simulink model "RaibertControl"  (R2022a)
settings: Solver=ode4  StartTime=0.0  StopTime=10  FixedStep=1/1000  RelTol=1e-3  AbsTol=1e-3  EnableMultiTasking=on
undefined symbols (not defined in the file or in its folder): Carrier, N, Ring, T, X, Y, Z
libraries: sm_lib x133, nesl_utility x25, Multibody_Parts_Lib x4, fl_lib x4
(part 7 of 7)

== matlab function RaibertControl/Final/Impedance Control1/to_dPolar ==
  data: theta1 input; theta2 input; dr output; dphi output; dtheta1 input; dtheta2 input
function [dr,dphi] = Velocity(theta1,theta2,dtheta1,dtheta2)
%VELOCITY
%    [DR,DPHI] = VELOCITY(THETA1,THETA2,DTHETA1,DTHETA2)

%    This function was generated by the Symbolic Math Toolbox version 8.6.
%    17-May-2022 09:32:08

dr = dtheta1.*(sin(acos(sqrt((sin(theta1-pi./2.0).*(7.0./4.0e+1)+sin(theta2+pi./2.0).*(7.0./4.0e+1)).^2+abs(cos(theta1-pi./2.0).*(7.0./4.0e+1)+cos(theta2+pi./2.0).*(7.0./4.0e+1)+3.0./2.5e+1).^2).*(5.0./3.0))+atan2(sin(theta1-pi./2.0).*(-7.0./4.0e+1)-sin(theta2+pi./2.0).*(7.0./4.0e+1),abs(cos(theta1-pi./2.0).*(7.0./4.0e+1)+cos(theta2+pi./2.0).*(7.0./4.0e+1)+3.0./2.5e+1))+6.012387278395987e-2).*(1.0./sqrt((sin(theta1-pi./2.0).*(7.0./4.0e+1)+sin(theta2+pi./2.0).*(7.0./4.0e+1)).^2+abs(cos(theta1-pi./2.0).*(7.0./4.0e+1)+cos(theta2+pi./2.0).*(7.0./4.0e+1)+3.0./2.5e+1).^2).*(cos(theta1-pi./2.0).*(sin(theta1-pi./2.0).*(7.0./4.0e+1)+sin(theta2+pi./2.0).*(7.0./4.0e+1)).*(7.0./2.0e+1)-abs(cos(theta1-pi./2.0).*(7.0./4.0e+1)+cos(theta2+pi./2.0).*(7.0./4.0e+1)+3.0./2.5e+1).*sign(cos(theta1-pi./2.0).*(7.0./4.0e+1)+cos(theta2+pi./2.0).*(7.0./4.0e+1)+3.0./2.5e+1).*sin(theta1-pi./2.0).*(7.0./2.0e+1)).*1.0./sqrt((sin(theta1-pi./2.0).*(7.0./4.0e+1)+sin(theta2+pi./2.0).*(7.0./4.0e+1)).^2.*(-2.5e+1./9.0)-abs(cos(theta1-pi./2.0).*(7.0./4.0e+1)+cos(theta2+pi./2.0).*(7.0./4.0e+1)+3.0./2.5e+1).^2.*(2.5e+1./9.0)+1.0).*(5.0./6.0)+(abs(cos(theta1-pi./2.0).*(7.0./4.0e+1)+cos(theta2+pi./2.0).*(7.0./4.0e+1)+3.0./2.5e+1).^2.*((cos(theta1-pi./2.0).*(7.0./4.0e+1))./abs(cos(theta1-pi./2.0).*(7.0./4.0e+1)+cos(theta2+pi./2.0).*(7.0./4.0e+1)+3.0./2.5e+1)+1.0./abs(cos(theta1-pi./2.0).*(7.0./4.0e+1)+cos(theta2+pi./2.0).*(7.0./4.0e+1)+3.0./2.5e+1).^2.*sign(cos(theta1-pi./2.0).*(7.0./4.0e+1)+cos(theta2+pi./2.0).*(7.0./4.0e+1)+3.0./2.5e+1).*sin(theta1-pi./2.0).*(sin(theta1-pi./2.0).*(7.0./4.0e+1)+sin(theta2+pi./2.0).*(7.0./4.0e+1)).*(7.0./4.0e+1)))./((sin(theta1-pi./2.0).*(7.0./4.0e+1)+sin(theta2+pi./2.0).*(7.0./4.0e+1)).^2+abs(cos(theta1-pi./2.0).*(7.0./4.0e+1)+cos(theta2+pi./2.0).*(7.0./4.0e+1)+3.0./2.5e+1).^2)).*(cos(acos(sqrt((sin(theta1-pi./2.0).*(7.0./4.0e+1)+sin(theta2+pi./2.0).*(7.0./4.0e+1)).^2+abs(cos(theta1-pi./2.0).*(7.0./4.0e+1)+cos(theta2+pi./2.0).*(7.0./4.0e+1)+3.0./2.5e+1).^2).*(5.0./3.0))+atan2(sin(theta1-pi./2.0).*(-7.0./4.0e+1)-sin(theta2+pi./2.0).*(7.0./4.0e+1),abs(cos(theta1-pi./2.0).*(7.0./4.0e+1)+cos(theta2+pi./2.0).*(7.0./4.0e+1)+3.0./2.5e+1))+6.012387278395987e-2).*(-3.328470665197855e-1)+cos(theta2+pi./2.0).*(7.0./4.0e+1)+3.0./5.0e+1).*6.65694133039571e-1+cos(acos(sqrt((sin(theta1-pi./2.0).*(7.0./4.0e+1)+sin(theta2+pi./2.0).*(7.0./4.0e+1)).^2+abs(cos(theta1-pi./2.0).*(7.0./4.0e+1)+cos(theta2+pi./2.0).*(7.0./4.0e+1)+3.0./2.5e+1).^2).*(5.0./3.0))+atan2(sin(theta1-pi./2.0).*(-7.0./4.0e+1)-sin(theta2+pi./2.0).*(7.0./4.0e+1),abs(cos(theta1-pi./2.0).*(7.0./4.0e+1)+cos(theta2+pi./2.0).*(7.0./4.0e+1)+3.0./2.5e+1))+6.012387278395987e-2).*(sin(acos(sqrt((sin(theta1-pi./2.0).*(7.0./4.0e+1)+sin(theta2+pi./2.0).*(7.0./4.0e+1)).^2+abs(cos(theta1-pi./2.0).*(7.0./4.0e+1)+cos(theta2+pi./2.0).*(7.0./4.0e+1)+3.0./2.5e+1).^2).*(5.0./3.0))+atan2(sin(theta1-pi./2.0).*(-7.0./4.0e+1)-sin(theta2+pi./2.0).*(7.0./4.0e+1),abs(cos(theta1-pi./2.0).*(7.0./4.0e+1)+cos(theta2+pi./2.0).*(7.0./4.0e+1)+3.0./2.5e+1))+6.012387278395987e-2).*3.328470665197855e-1+sin(theta2+pi./2.0).*(7.0./4.0e+1)).*(1.0./sqrt((sin(theta1-pi./2.0).*(7.0./4.0e+1)+sin(theta2+pi./2.0).*(7.0./4.0e+1)).^2+abs(cos(theta1-pi./2.0).*(7.0./4.0e+1)+cos(theta2+pi./2.0).*(7.0./4.0e+1)+3.0./2.5e+1).^2).*(cos(theta1-pi./2.0).*(sin(theta1-pi./2.0).*(7.0./4.0e+1)+sin(theta2+pi./2.0).*(7.0./4.0e+1)).*(7.0./2.0e+1)-abs(cos(theta1-pi./2.0).*(7.0./4.0e+1)+cos(theta2+pi./2.0).*(7.0./4.0e+1)+3.0./2.5e+1).*sign(cos(theta1-pi./2.0).*(7.0./4.0e+1)+cos(theta2+pi./2.0).*(7.0./4.0e+1)+3.0./2.5e+1).*sin(theta1-pi./2.0).*(7.0./2.0e+1)).*1.0./sqrt((sin(theta1-pi./2.0).*(7.0./4.0e+1)+sin(theta2+pi./2.0).*(7.0./4.0e+1)).^2.*(-2.5e+1./9.0)-abs(cos(theta1-pi./2.0).*(7.0./4.0e+1)+cos(theta2+pi./2.0).*(7.0./4.0e+1)+3.0./2.5e+1).^2.*(2.5e+1./9.0)+1.0).*(5.0./6.0)+(abs(cos(theta1-pi./2.0).*(7.0./4.0e+1)+cos(theta2+pi./2.0).*(7.0./4.0e+1)+3.0./2.5e+1).^2.*((cos(theta1-pi./2.0).*(7.0./4.0e+1))./abs(cos(theta1-pi./2.0).*(7.0./4.0e+1)+cos(theta2+pi./2.0).*(7.0./4.0e+1)+3.0./2.5e+1)+1.0./abs(cos(theta1-pi./2.0).*(7.0./4.0e+1)+cos(theta2+pi./2.0).*(7.0./4.0e+1)+3.0./2.5e+1).^2.*sign(cos(theta1-pi./2.0).*(7.0./4.0e+1)+cos(theta2+pi./2.0).*(7.0./4.0e+1)+3.0./2.5e+1).*sin(theta1-pi./2.0).*(sin(theta1-pi./2.0).*(7.0./4.0e+1)+sin(theta2+pi./2.0).*(7.0./4.0e+1)).*(7.0./4.0e+1)))./((sin(theta1-pi./2.0).*(7.0./4.0e+1)+sin(theta2+pi./2.0).*(7.0./4.0e+1)).^2+abs(cos(theta1-pi./2.0).*(7.0./4.0e+1)+cos(theta2+pi./2.0).*(7.0./4.0e+1)+3.0./2.5e+1).^2)).*6.65694133039571e-1).*1.0./sqrt((cos(acos(sqrt((sin(theta1-pi./2.0).*(7.0./4.0e+1)+sin(theta2+pi./2.0).*(7.0./4.0e+1)).^2+abs(cos(theta1-pi./2.0).*(7.0./4.0e+1)+cos(theta2+pi./2.0).*(7.0./4.0e+1)+3.0./2.5e+1).^2).*(5.0./3.0))+atan2(sin(theta1-pi./2.0).*(-7.0./4.0e+1)-sin(theta2+pi./2.0).*(7.0./4.0e+1),abs(cos(theta1-pi./2.0).*(7.0./4.0e+1)+cos(theta2+pi./2.0).*(7.0./4.0e+1)+3.0./2.5e+1))+6.012387278395987e-2).*(-3.328470665197855e-1)+cos(theta2+pi./2.0).*(7.0./4.0e+1)+3.0./5.0e+1).^2+(sin(acos(sqrt((sin(theta1-pi./2.0).*(7.0./4.0e+1)+sin(theta2+pi./2.0).*(7.0./4.0e+1)).^2+abs(cos(theta1-pi./2.0).*(7.0./4.0e+1)+cos(theta2+pi./2.0).*(7.0./4.0e+1)+3.0./2.5e+1).^2).*(5.0./3.0))+atan2(sin(theta1-pi./2.0).*(-7.0./4.0e+1)-sin(theta2+pi./2.0).*(7.0./4.0e+1),abs(cos(theta1-pi./2.0).*(7.0./4.0e+1)+cos(theta2+pi./2.0).*(7.0./4.0e+1)+3.0./2.5e+1))+6.012387278395987e-2).*3.328470665197855e-1+sin(theta2+pi./2.0).*(7.0./4.0e+1)).^2).*(-1.0./2.0)+(dtheta2.*((sin(acos(sqrt((sin(theta1-pi./2.0).*(7.0./4.0e+1)+sin(theta2+pi./2.0).*(7.0./4.0e+1)).^2+abs(cos(theta1-pi./2.0).*(7.0./4.0e+1)+cos(theta2+pi./2.0).*(7.0./4.0e+1)+3.0./2.5e+1).^2).*(5.0./3.0))+atan2(sin(theta1-pi./2.0).*(-7.0./4.0e+1)-sin(theta2+pi./2.0).*(7.0./4.0e+1),abs(cos(theta1-pi./2.0).*(7.0./4.0e+1)+cos(theta2+pi./2.0).*(7.0./4.0e+1)+3.0./2.5e+1))+6.012387278395987e-2).*3.328470665197855e-1+sin(theta2+pi./2.0).*(7.0./4.0e+1)).*(cos(theta2+pi./2.0).*(7.0./4.0e+1)-cos(acos(sqrt((sin(theta1-pi./2.0).*(7.0./4.0e+1)+sin(theta2+pi./2.0).*(7.0./4.0e+1)).^2+abs(cos(theta1-pi./2.0).*(7.0./4.0e+1)+cos(theta2+pi./2.0).*(7.0./4.0e+1)+3.0./2.5e+1).^2).*(5.0./3.0))+atan2(sin(theta1-pi./2.0).*(-7.0./4.0e+1)-sin(theta2+pi./2.0).*(7.0./4.0e+1),abs(cos(theta1-pi./2.0).*(7.0./4.0e+1)+cos(theta2+pi./2.0).*(7.0./4.0e+1)+3.0./2.5e+1))+6.012387278395987e-2).*(1.0./sqrt((sin(theta1-pi./2.0).*(7.0./4.0e+1)+sin(theta2+pi./2.0).*(7.0./4.0e+1)).^2+abs(cos(theta1-pi./2.0).*(7.0./4.0e+1)+cos(theta2+pi./2.0).*(7.0./4.0e+1)+3.0./2.5e+1).^2).*(cos(theta2+pi./2.0).*(sin(theta1-pi./2.0).*(7.0./4.0e+1)+sin(theta2+pi./2.0).*(7.0./4.0e+1)).*(7.0./2.0e+1)-abs(cos(theta1-pi./2.0).*(7.0./4.0e+1)+cos(theta2+pi./2.0).*(7.0./4.0e+1)+3.0./2.5e+1).*sign(cos(theta1-pi./2.0).*(7.0./4.0e+1)+cos(theta2+pi./2.0).*(7.0./4.0e+1)+3.0./2.5e+1).*sin(theta2+pi./2.0).*(7.0./2.0e+1)).*1.0./sqrt((sin(theta1-pi./2.0).*(7.0./4.0e+1)+sin(theta2+pi./2.0).*(7.0./4.0e+1)).^2.*(-2.5e+1./9.0)-abs(cos(theta1-pi./2.0).*(7.0./4.0e+1)+cos(theta2+pi./2.0).*(7.0./4.0e+1)+3.0./2.5e+1).^2.*(2.5e+1./9.0)+1.0).*(5.0./6.0)+(abs(cos(theta1-pi./2.0).*(7.0./4.0e+1)+cos(theta2+pi./2.0).*(7.0./4.0e+1)+3.0./2.5e+1).^2.*((cos(theta2+pi./2.0).*(7.0./4.0e+1))./abs(cos(theta1-pi./2.0).*(7.0./4.0e+1)+cos(theta2+pi./2.0).*(7.0./4.0e+1)+3.0./2.5e+1)+1.0./abs(cos(theta1-pi./2.0).*(7.0./4.0e+1)+cos(theta2+pi./2.0).*(7.0./4.0e+1)+3.0./2.5e+1).^2.*sign(cos(theta1-pi./2.0).*(7.0./4.0e+1)+cos(theta2+pi./2.0).*(7.0./4.0e+1)+3.0./2.5e+1).*sin(theta2+pi./2.0).*(sin(theta1-pi./2.0).*(7.0./4.0e+1)+sin(theta2+pi./2.0).*(7.0./4.0e+1)).*(7.0./4.0e+1)))./((sin(theta1-pi./2.0).*(7.0./4.0e+1)+sin(theta2+pi./2.0).*(7.0./4.0e+1)).^2+abs(cos(theta1-pi./2.0).*(7.0./4.0e+1)+cos(theta2+pi./2.0).*(7.0./4.0e+1)+3.0./2.5e+1).^2)).*3.328470665197855e-1).*2.0-(sin(theta2+pi./2.0).*(7.0./4.0e+1)+sin(acos(sqrt((sin(theta1-pi./2.0).*(7.0./4.0e+1)+sin(theta2+pi./2.0).*(7.0./4.0e+1)).^2+abs(cos(theta1-pi./2.0).*(7.0./4.0e+1)+cos(theta2+pi./2.0).*(7.0./4.0e+1)+3.0./2.5e+1).^2).*(5.0./3.0))+atan2(sin(theta1-pi./2.0).*(-7.0./4.0e+1)-sin(theta2+pi./2.0).*(7.0./4.0e+1),abs(cos(theta1-pi./2.0).*(7.0./4.0e+1)+cos(theta2+pi./2.0).*(7.0./4.0e+1)+3.0./2.5e+1))+6.012387278395987e-2).*(1.0./sqrt((sin(theta1-pi./2.0).*(7.0./4.0e+1)+sin(theta2+pi./2.0).*(7.0./4.0e+1)).^2+abs(cos(theta1-pi./2.0).*(7.0./4.0e+1)+cos(theta2+pi./2.0).*(7.0./4.0e+1)+3.0./2.5e+1).^2).*(cos(theta2+pi./2.0).*(sin(theta1-pi./2.0).*(7.0./4.0e+1)+sin(theta2+pi./2.0).*(7.0./4.0e+1)).*(7.0./2.0e+1)-abs(cos(theta1-pi./2.0).*(7.0./4.0e+1)+cos(theta2+pi./2.0).*(7.0./4.0e+1)+3.0./2.5e+1).*sign(cos(theta1-pi./2.0).*(7.0./4.0e+1)+cos(theta2+pi./2.0).*(7.0./4.0e+1)+3.0./2.5e+1).*sin(theta2+pi./2.0).*(7.0./2.0e+1)).*1.0./sqrt((sin(theta1-pi./2.0).*(7.0./4.0e+1)+sin(theta2+pi./2.0).*(7.0./4.0e+1)).^2.*(-2.5e+1./9.0)-abs(cos(theta1-pi./2.0).*(7.0./4.0e+1)+cos(theta2+pi./2.0).*(7.0./4.0e+1)+3.0./2.5e+1).^2.*(2.5e+1./9.0)+1.0).*(5.0./6.0)+(abs(cos(theta1-pi./2.0).*(7.0./4.0e+1)+cos(theta2+pi./2.0).*(7.0./4.0e+1)+3.0./2.5e+1).^2.*((cos(theta2+pi./2.0).*(7.0./4.0e+1))./abs(cos(theta1-pi./2.0).*(7.0./4.0e+1)+cos(theta2+pi./2.0).*(7.0./4.0e+1)+3.0./2.5e+1)+1.0./abs(cos(theta1-pi./2.0).*(7.0./4.0e+1)+cos(theta2+pi./2.0).*(7.0./4.0e+1)+3.0./2.5e+1).^2.*sign(cos(theta1-pi./2.0).*(7.0./4.0e+1)+cos(theta2+pi./2.0).*(7.0./4.0e+1)+3.0./2.5e+1).*sin(theta2+pi./2.0).*(sin(theta1-pi./2.0).*(7.0./4.0e+1)+sin(theta2+pi./2.0).*(7.0./4.0e+1)).*(7.0./4.0e+1)))./((sin(theta1-pi./2.0).*(7.0./4.0e+1)+sin(theta2+pi./2.0).*(7.0./4.0e+1)).^2+abs(cos(theta1-pi./2.0).*(7.0./4.0e+1)+cos(theta2+pi./2.0).*(7.0./4.0e+1)+3.0./2.5e+1).^2)).*3.328470665197855e-1).*(cos(acos(sqrt((sin(theta1-pi./2.0).*(7.0./4.0e+1)+sin(theta2+pi./2.0).*(7.0./4.0e+1)).^2+abs(cos(theta1-pi./2.0).*(7.0./4.0e+1)+cos(theta2+pi./2.0).*(7.0./4.0e+1)+3.0./2.5e+1).^2).*(5.0./3.0))+atan2(sin(theta1-pi./2.0).*(-7.0./4.0e+1)-sin(theta2+pi./2.0).*(7.0./4.0e+1),abs(cos(theta1-pi./2.0).*(7.0./4.0e+1)+cos(theta2+pi./2.0).*(7.0./4.0e+1)+3.0./2.5e+1))+6.012387278395987e-2).*(-3.328470665197855e-1)+cos(theta2+pi./2.0).*(7.0./4.0e+1)+3.0./5.0e+1).*2.0).*1.0./sqrt((cos(acos(sqrt((sin(theta1-pi./2.0).*(7.0./4.0e+1)+sin(theta2+pi./2.0).*(7.0./4.0e+1)).^2+abs(cos(theta1-pi./2.0).*(7.0./4.0e+1)+cos(theta2+pi./2.0).*(7.0./4.0e+1)+3.0./2.5e+1).^2).*(5.0./3.0))+atan2(sin(theta1-pi./2.0).*(-7.0./4.0e+1)-sin(theta2+pi./2.0).*(7.0./4.0e+1),abs(cos(theta1-pi./2.0).*(7.0./4.0e+1)+cos(theta2+pi./2.0).*(7.0./4.0e+1)+3.0./2.5e+1))+6.012387278395987e-2).*(-3.328470665197855e-1)+cos(theta2+pi./2.0).*(7.0./4.0e+1)+3.0./5.0e+1).^2+(sin(acos(sqrt((sin(theta1-pi./2.0).*(7.0./4.0e+1)+sin(theta2+pi./2.0).*(7.0./4.0e+1)).^2+abs(cos(theta1-pi./2.0).*(7.0./4.0e+1)+cos(theta2+pi./2.0).*(7.0./4.0e+1)+3.0./2.5e+1).^2).*(5.0./3.0))+atan2(sin(theta1-pi./2.0).*(-7.0./4.0e+1)-sin(theta2+pi./2.0).*(7.0./4.0e+1),abs(cos(theta1-pi./2.0).*(7.0./4.0e+1)+cos(theta2+pi./2.0).*(7.0./4.0e+1)+3.0./2.5e+1))+6.012387278395987e-2).*3.328470665197855e-1+sin(theta2+pi./2.0).*(7.0./4.0e+1)).^2))./2.0;
if nargout > 1
    dphi = (dtheta1.*((cos(acos(sqrt((sin(theta1-pi./2.0).*(7.0./4.0e+1)+sin(theta2+pi./2.0).*(7.0./4.0e+1)).^2+abs(cos(theta1-pi./2.0).*(7.0./4.0e+1)+cos(theta2+pi./2.0).*(7.0./4.0e+1)+3.0./2.5e+1).^2).*(5.0./3.0))+atan2(sin(theta1-pi./2.0).*(-7.0./4.0e+1)-sin(theta2+pi./2.0).*(7.0./4.0e+1),abs(cos(theta1-pi./2.0).*(7.0./4.0e+1)+cos(theta2+pi./2.0).*(7.0./4.0e+1)+3.0./2.5e+1))+6.012387278395987e-2).*(1.0./sqrt((sin(theta1-pi./2.0).*(7.0./4.0e+1)+sin(theta2+pi./2.0).*(7.0./4.0e+1)).^2+abs(cos(theta1-pi./2.0).*(7.0./4.0e+1)+cos(theta2+pi./2.0).*(7.0./4.0e+1)+3.0./2.5e+1).^2).*(cos(theta1-pi./2.0).*(sin(theta1-pi./2.0).*(7.0./4.0e+1)+sin(theta2+pi./2.0).*(7.0./4.0e+1)).*(7.0./2.0e+1)-abs(cos(theta1-pi./2.0).*(7.0./4.0e+1)+cos(theta2+pi./2.0).*(7.0./4.0e+1)+3.0./2.5e+1).*sign(cos(theta1-pi./2.0).*(7.0./4.0e+1)+cos(theta2+pi./2.0).*(7.0./4.0e+1)+3.0./2.5e+1).*sin(theta1-pi./2.0).*(7.0./2.0e+1)).*1.0./sqrt((sin(theta1-pi./2.0).*(7.0./4.0e+1)+sin(theta2+pi./2.0).*(7.0./4.0e+1)).^2.*(-2.5e+1./9.0)-abs(cos(theta1-pi./2.0).*(7.0./4.0e+1)+cos(theta2+pi./2.0).*(7.0./4.0e+1)+3.0./2.5e+1).^2.*(2.5e+1./9.0)+1.0).*(5.0./6.0)+(abs(cos(theta1-pi./2.0).*(7.0./4.0e+1)+cos(theta2+pi./2.0).*(7.0./4.0e+1)+3.0./2.5e+1).^2.*((cos(theta1-pi./2.0).*(7.0./4.0e+1))./abs(cos(theta1-pi./2.0).*(7.0./4.0e+1)+cos(theta2+pi./2.0).*(7.0./4.0e+1)+3.0./2.5e+1)+1.0./abs(cos(theta1-pi./2.0).*(7.0./4.0e+1)+cos(theta2+pi./2.0).*(7.0./4.0e+1)+3.0./2.5e+1).^2.*sign(cos(theta1-pi./2.0).*(7.0./4.0e+1)+cos(theta2+pi./2.0).*(7.0./4.0e+1)+3.0./2.5e+1).*sin(theta1-pi./2.0).*(sin(theta1-pi./2.0).*(7.0./4.0e+1)+sin(theta2+pi./2.0).*(7.0./4.0e+1)).*(7.0./4.0e+1)))./((sin(theta1-pi./2.0).*(7.0./4.0e+1)+sin(theta2+pi./2.0).*(7.0./4.0e+1)).^2+abs(cos(theta1-pi./2.0).*(7.0./4.0e+1)+cos(theta2+pi./2.0).*(7.0./4.0e+1)+3.0./2.5e+1).^2)).*3.328470665197855e-1)./(cos(acos(sqrt((sin(theta1-pi./2.0).*(7.0./4.0e+1)+sin(theta2+pi./2.0).*(7.0./4.0e+1)).^2+abs(cos(theta1-pi./2.0).*(7.0./4.0e+1)+cos(theta2+pi./2.0).*(7.0./4.0e+1)+3.0./2.5e+1).^2).*(5.0./3.0))+atan2(sin(theta1-pi./2.0).*(-7.0./4.0e+1)-sin(theta2+pi./2.0).*(7.0./4.0e+1),abs(cos(theta1-pi./2.0).*(7.0./4.0e+1)+cos(theta2+pi./2.0).*(7.0./4.0e+1)+3.0./2.5e+1))+6.012387278395987e-2).*(-3.328470665197855e-1)+cos(theta2+pi./2.0).*(7.0./4.0e+1)+3.0./5.0e+1)-sin(acos(sqrt((sin(theta1-pi./2.0).*(7.0./4.0e+1)+sin(theta2+pi./2.0).*(7.0./4.0e+1)).^2+abs(cos(theta1-pi./2.0).*(7.0./4.0e+1)+cos(theta2+pi./2.0).*(7.0./4.0e+1)+3.0./2.5e+1).^2).*(5.0./3.0))+atan2(sin(theta1-pi./2.0).*(-7.0./4.0e+1)-sin(theta2+pi./2.0).*(7.0./4.0e+1),abs(cos(theta1-pi./2.0).*(7.0./4.0e+1)+cos(theta2+pi./2.0).*(7.0./4.0e+1)+3.0./2.5e+1))+6.012387278395987e-2).*(sin(acos(sqrt((sin(theta1-pi./2.0).*(7.0./4.0e+1)+sin(theta2+pi./2.0).*(7.0./4.0e+1)).^2+abs(cos(theta1-pi./2.0).*(7.0./4.0e+1)+cos(theta2+pi./2.0).*(7.0./4.0e+1)+3.0./2.5e+1).^2).*(5.0./3.0))+atan2(sin(theta1-pi./2.0).*(-7.0./4.0e+1)-sin(theta2+pi./2.0).*(7.0./4.0e+1),abs(cos(theta1-pi./2.0).*(7.0./4.0e+1)+cos(theta2+pi./2.0).*(7.0./4.0e+1)+3.0./2.5e+1))+6.012387278395987e-2).*3.328470665197855e-1+sin(theta2+pi./2.0).*(7.0./4.0e+1)).*(1.0./sqrt((sin(theta1-pi./2.0).*(7.0./4.0e+1)+sin(theta2+pi./2.0).*(7.0./4.0e+1)).^2+abs(cos(theta1-pi./2.0).*(7.0./4.0e+1)+cos(theta2+pi./2.0).*(7.0./4.0e+1)+3.0./2.5e+1).^2).*(cos(theta1-pi./2.0).*(sin(theta1-pi./2.0).*(7.0./4.0e+1)+sin(theta2+pi./2.0).*(7.0./4.0e+1)).*(7.0./2.0e+1)-abs(cos(theta1-pi./2.0).*(7.0./4.0e+1)+cos(theta2+pi./2.0).*(7.0./4.0e+1)+3.0./2.5e+1).*sign(cos(theta1-pi./2.0).*(7.0./4.0e+1)+cos(theta2+pi./2.0).*(7.0./4.0e+1)+3.0./2.5e+1).*sin(theta1-pi./2.0).*(7.0./2.0e+1)).*1.0./sqrt((sin(theta1-pi./2.0).*(7.0./4.0e+1)+sin(theta2+pi./2.0).*(7.0./4.0e+1)).^2.*(-2.5e+1./9.0)-abs(cos(theta1-pi./2.0).*(7.0./4.0e+1)+cos(theta2+pi./2.0).*(7.0./4.0e+1)+3.0./2.5e+1).^2.*(2.5e+1./9.0)+1.0).*(5.0./6.0)+(abs(cos(theta1-pi./2.0).*(7.0./4.0e+1)+cos(theta2+pi./2.0).*(7.0./4.0e+1)+3.0./2.5e+1).^2.*((cos(theta1-pi./2.0).*(7.0./4.0e+1))./abs(cos(theta1-pi./2.0).*(7.0./4.0e+1)+cos(theta2+pi./2.0).*(7.0./4.0e+1)+3.0./2.5e+1)+1.0./abs(cos(theta1-pi./2.0).*(7.0./4.0e+1)+cos(theta2+pi./2.0).*(7.0./4.0e+1)+3.0./2.5e+1).^2.*sign(cos(theta1-pi./2.0).*(7.0./4.0e+1)+cos(theta2+pi./2.0).*(7.0./4.0e+1)+3.0./2.5e+1).*sin(theta1-pi./2.0).*(sin(theta1-pi./2.0).*(7.0./4.0e+1)+sin(theta2+pi./2.0).*(7.0./4.0e+1)).*(7.0./4.0e+1)))./((sin(theta1-pi./2.0).*(7.0./4.0e+1)+sin(theta2+pi./2.0).*(7.0./4.0e+1)).^2+abs(cos(theta1-pi./2.0).*(7.0./4.0e+1)+cos(theta2+pi./2.0).*(7.0./4.0e+1)+3.0./2.5e+1).^2)).*1.0./(cos(acos(sqrt((sin(theta1-pi./2.0).*(7.0./4.0e+1)+sin(theta2+pi./2.0).*(7.0./4.0e+1)).^2+abs(cos(theta1-pi./2.0).*(7.0./4.0e+1)+cos(theta2+pi./2.0).*(7.0./4.0e+1)+3.0./2.5e+1).^2).*(5.0./3.0))+atan2(sin(theta1-pi./2.0).*(-7.0./4.0e+1)-sin(theta2+pi./2.0).*(7.0./4.0e+1),abs(cos(theta1-pi./2.0).*(7.0./4.0e+1)+cos(theta2+pi./2.0).*(7.0./4.0e+1)+3.0./2.5e+1))+6.012387278395987e-2).*(-3.328470665197855e-1)+cos(theta2+pi./2.0).*(7.0./4.0e+1)+3.0./5.0e+1).^2.*3.328470665197855e-1).*(cos(acos(sqrt((sin(theta1-pi./2.0).*(7.0./4.0e+1)+sin(theta2+pi./2.0).*(7.0./4.0e+1)).^2+abs(cos(theta1-pi./2.0).*(7.0./4.0e+1)+cos(theta2+pi./2.0).*(7.0./4.0e+1)+3.0./2.5e+1).^2).*(5.0./3.0))+atan2(sin(theta1-pi./2.0).*(-7.0./4.0e+1)-sin(theta2+pi./2.0).*(7.0./4.0e+1),abs(cos(theta1-pi./2.0).*(7.0./4.0e+1)+cos(theta2+pi./2.0).*(7.0./4.0e+1)+3.0./2.5e+1))+6.012387278395987e-2).*(-3.328470665197855e-1)+cos(theta2+pi./2.0).*(7.0./4.0e+1)+3.0./5.0e+1).^2)./((cos(acos(sqrt((sin(theta1-pi./2.0).*(7.0./4.0e+1)+sin(theta2+pi./2.0).*(7.0./4.0e+1)).^2+abs(cos(theta1-pi./2.0).*(7.0./4.0e+1)+cos(theta2+pi./2.0).*(7.0./4.0e+1)+3.0./2.5e+1).^2).*(5.0./3.0))+atan2(sin(theta1-pi./2.0).*(-7.0./4.0e+1)-sin(theta2+pi./2.0).*(7.0./4.0e+1),abs(cos(theta1-pi./2.0).*(7.0./4.0e+1)+cos(theta2+pi./2.0).*(7.0./4.0e+1)+3.0./2.5e+1))+6.012387278395987e-2).*(-3.328470665197855e-1)+cos(theta2+pi./2.0).*(7.0./4.0e+1)+3.0./5.0e+1).^2+(sin(acos(sqrt((sin(theta1-pi./2.0).*(7.0./4.0e+1)+sin(theta2+pi./2.0).*(7.0./4.0e+1)).^2+abs(cos(theta1-pi./2.0).*(7.0./4.0e+1)+cos(theta2+pi./2.0).*(7.0./4.0e+1)+3.0./2.5e+1).^2).*(5.0./3.0))+atan2(sin(theta1-pi./2.0).*(-7.0./4.0e+1)-sin(theta2+pi./2.0).*(7.0./4.0e+1),abs(cos(theta1-pi./2.0).*(7.0./4.0e+1)+cos(theta2+pi./2.0).*(7.0./4.0e+1)+3.0./2.5e+1))+6.012387278395987e-2).*3.328470665197855e-1+sin(theta2+pi./2.0).*(7.0./4.0e+1)).^2)-(dtheta2.*((cos(theta2+pi./2.0).*(7.0./4.0e+1)-cos(acos(sqrt((sin(theta1-pi./2.0).*(7.0./4.0e+1)+sin(theta2+pi./2.0).*(7.0./4.0e+1)).^2+abs(cos(theta1-pi./2.0).*(7.0./4.0e+1)+cos(theta2+pi./2.0).*(7.0./4.0e+1)+3.0./2.5e+1).^2).*(5.0./3.0))+atan2(sin(theta1-pi./2.0).*(-7.0./4.0e+1)-sin(theta2+pi./2.0).*(7.0./4.0e+1),abs(cos(theta1-pi./2.0).*(7.0./4.0e+1)+cos(theta2+pi./2.0).*(7.0./4.0e+1)+3.0./2.5e+1))+6.012387278395987e-2).*(1.0./sqrt((sin(theta1-pi./2.0).*(7.0./4.0e+1)+sin(theta2+pi./2.0).*(7.0./4.0e+1)).^2+abs(cos(theta1-pi./2.0).*(7.0./4.0e+1)+cos(theta2+pi./2.0).*(7.0./4.0e+1)+3.0./2.5e+1).^2).*(cos(theta2+pi./2.0).*(sin(theta1-pi./2.0).*(7.0./4.0e+1)+sin(theta2+pi./2.0).*(7.0./4.0e+1)).*(7.0./2.0e+1)-abs(cos(theta1-pi./2.0).*(7.0./4.0e+1)+cos(theta2+pi./2.0).*(7.0./4.0e+1)+3.0./2.5e+1).*sign(cos(theta1-pi./2.0).*(7.0./4.0e+1)+cos(theta2+pi./2.0).*(7.0./4.0e+1)+3.0./2.5e+1).*sin(theta2+pi./2.0).*(7.0./2.0e+1)).*1.0./sqrt((sin(theta1-pi./2.0).*(7.0./4.0e+1)+sin(theta2+pi./2.0).*(7.0./4.0e+1)).^2.*(-2.5e+1./9.0)-abs(cos(theta1-pi./2.0).*(7.0./4.0e+1)+cos(theta2+pi./2.0).*(7.0./4.0e+1)+3.0./2.5e+1).^2.*(2.5e+1./9.0)+1.0).*(5.0./6.0)+(abs(cos(theta1-pi./2.0).*(7.0./4.0e+1)+cos(theta2+pi./2.0).*(7.0./4.0e+1)+3.0./2.5e+1).^2.*((cos(theta2+pi./2.0).*(7.0./4.0e+1))./abs(cos(theta1-pi./2.0).*(7.0./4.0e+1)+cos(theta2+pi./2.0).*(7.0./4.0e+1)+3.0./2.5e+1)+1.0./abs(cos(theta1-pi./2.0).*(7.0./4.0e+1)+cos(theta2+pi./2.0).*(7.0./4.0e+1)+3.0./2.5e+1).^2.*sign(cos(theta1-pi./2.0).*(7.0./4.0e+1)+cos(theta2+pi./2.0).*(7.0./4.0e+1)+3.0./2.5e+1).*sin(theta2+pi./2.0).*(sin(theta1-pi./2.0).*(7.0./4.0e+1)+sin(theta2+pi./2.0).*(7.0./4.0e+1)).*(7.0./4.0e+1)))./((sin(theta1-pi./2.0).*(7.0./4.0e+1)+sin(theta2+pi./2.0).*(7.0./4.0e+1)).^2+abs(cos(theta1-pi./2.0).*(7.0./4.0e+1)+cos(theta2+pi./2.0).*(7.0./4.0e+1)+3.0./2.5e+1).^2)).*3.328470665197855e-1)./(cos(acos(sqrt((sin(theta1-pi./2.0).*(7.0./4.0e+1)+sin(theta2+pi./2.0).*(7.0./4.0e+1)).^2+abs(cos(theta1-pi./2.0).*(7.0./4.0e+1)+cos(theta2+pi./2.0).*(7.0./4.0e+1)+3.0./2.5e+1).^2).*(5.0./3.0))+atan2(sin(theta1-pi./2.0).*(-7.0./4.0e+1)-sin(theta2+pi./2.0).*(7.0./4.0e+1),abs(cos(theta1-pi./2.0).*(7.0./4.0e+1)+cos(theta2+pi./2.0).*(7.0./4.0e+1)+3.0./2.5e+1))+6.012387278395987e-2).*(-3.328470665197855e-1)+cos(theta2+pi./2.0).*(7.0./4.0e+1)+3.0./5.0e+1)+(sin(acos(sqrt((sin(theta1-pi./2.0).*(7.0./4.0e+1)+sin(theta2+pi./2.0).*(7.0./4.0e+1)).^2+abs(cos(theta1-pi./2.0).*(7.0./4.0e+1)+cos(theta2+pi./2.0).*(7.0./4.0e+1)+3.0./2.5e+1).^2).*(5.0./3.0))+atan2(sin(theta1-pi./2.0).*(-7.0./4.0e+1)-sin(theta2+pi./2.0).*(7.0./4.0e+1),abs(cos(theta1-pi./2.0).*(7.0./4.0e+1)+cos(theta2+pi./2.0).*(7.0./4.0e+1)+3.0./2.5e+1))+6.012387278395987e-2).*3.328470665197855e-1+sin(theta2+pi./2.0).*(7.0./4.0e+1)).*(sin(theta2+pi./2.0).*(7.0./4.0e+1)+sin(acos(sqrt((sin(theta1-pi./2.0).*(7.0./4.0e+1)+sin(theta2+pi./2.0).*(7.0./4.0e+1)).^2+abs(cos(theta1-pi./2.0).*(7.0./4.0e+1)+cos(theta2+pi./2.0).*(7.0./4.0e+1)+3.0./2.5e+1).^2).*(5.0./3.0))+atan2(sin(theta1-pi./2.0).*(-7.0./4.0e+1)-sin(theta2+pi./2.0).*(7.0./4.0e+1),abs(cos(theta1-pi./2.0).*(7.0./4.0e+1)+cos(theta2+pi./2.0).*(7.0./4.0e+1)+3.0./2.5e+1))+6.012387278395987e-2).*(1.0./sqrt((sin(theta1-pi./2.0).*(7.0./4.0e+1)+sin(theta2+pi./2.0).*(7.0./4.0e+1)).^2+abs(cos(theta1-pi./2.0).*(7.0./4.0e+1)+cos(theta2+pi./2.0).*(7.0./4.0e+1)+3.0./2.5e+1).^2).*(cos(theta2+pi./2.0).*(sin(theta1-pi./2.0).*(7.0./4.0e+1)+sin(theta2+pi./2.0).*(7.0./4.0e+1)).*(7.0./2.0e+1)-abs(cos(theta1-pi./2.0).*(7.0./4.0e+1)+cos(theta2+pi./2.0).*(7.0./4.0e+1)+3.0./2.5e+1).*sign(cos(theta1-pi./2.0).*(7.0./4.0e+1)+cos(theta2+pi./2.0).*(7.0./4.0e+1)+3.0./2.5e+1).*sin(theta2+pi./2.0).*(7.0./2.0e+1)).*1.0./sqrt((sin(theta1-pi./2.0).*(7.0./4.0e+1)+sin(theta2+pi./2.0).*(7.0./4.0e+1)).^2.*(-2.5e+1./9.0)-abs(cos(theta1-pi./2.0).*(7.0./4.0e+1)+cos(theta2+pi./2.0).*(7.0./4.0e+1)+3.0./2.5e+1).^2.*(2.5e+1./9.0)+1.0).*(5.0./6.0)+(abs(cos(theta1-pi./2.0).*(7.0./4.0e+1)+cos(theta2+pi./2.0).*(7.0./4.0e+1)+3.0./2.5e+1).^2.*((cos(theta2+pi./2.0).*(7.0./4.0e+1))./abs(cos(theta1-pi./2.0).*(7.0./4.0e+1)+cos(theta2+pi./2.0).*(7.0./4.0e+1)+3.0./2.5e+1)+1.0./abs(cos(theta1-pi./2.0).*(7.0./4.0e+1)+cos(theta2+pi./2.0).*(7.0./4.0e+1)+3.0./2.5e+1).^2.*sign(cos(theta1-pi./2.0).*(7.0./4.0e+1)+cos(theta2+pi./2.0).*(7.0./4.0e+1)+3.0./2.5e+1).*sin(theta2+pi./2.0).*(sin(theta1-pi./2.0).*(7.0./4.0e+1)+sin(theta2+pi./2.0).*(7.0./4.0e+1)).*(7.0./4.0e+1)))./((sin(theta1-pi./2.0).*(7.0./4.0e+1)+sin(theta2+pi./2.0).*(7.0./4.0e+1)).^2+abs(cos(theta1-pi./2.0).*(7.0./4.0e+1)+cos(theta2+pi./2.0).*(7.0./4.0e+1)+3.0./2.5e+1).^2)).*3.328470665197855e-1).*1.0./(cos(acos(sqrt((sin(theta1-pi./2.0).*(7.0./4.0e+1)+sin(theta2+pi./2.0).*(7.0./4.0e+1)).^2+abs(cos(theta1-pi./2.0).*(7.0./4.0e+1)+cos(theta2+pi./2.0).*(7.0./4.0e+1)+3.0./2.5e+1).^2).*(5.0./3.0))+atan2(sin(theta1-pi./2.0).*(-7.0./4.0e+1)-sin(theta2+pi./2.0).*(7.0./4.0e+1),abs(cos(theta1-pi./2.0).*(7.0./4.0e+1)+cos(theta2+pi./2.0).*(7.0./4.0e+1)+3.0./2.5e+1))+6.012387278395987e-2).*(-3.328470665197855e-1)+cos(theta2+pi./2.0).*(7.0./4.0e+1)+3.0./5.0e+1).^2).*(cos(acos(sqrt((sin(theta1-pi./2.0).*(7.0./4.0e+1)+sin(theta2+pi./2.0).*(7.0./4.0e+1)).^2+abs(cos(theta1-pi./2.0).*(7.0./4.0e+1)+cos(theta2+pi./2.0).*(7.0./4.0e+1)+3.0./2.5e+1).^2).*(5.0./3.0))+atan2(sin(theta1-pi./2.0).*(-7.0./4.0e+1)-sin(theta2+pi./2.0).*(7.0./4.0e+1),abs(cos(theta1-pi./2.0).*(7.0./4.0e+1)+cos(theta2+pi./2.0).*(7.0./4.0e+1)+3.0./2.5e+1))+6.012387278395987e-2).*(-3.328470665197855e-1)+cos(theta2+pi./2.0).*(7.0./4.0e+1)+3.0./5.0e+1).^2)./((cos(acos(sqrt((sin(theta1-pi./2.0).*(7.0./4.0e+1)+sin(theta2+pi./2.0).*(7.0./4.0e+1)).^2+abs(cos(theta1-pi./2.0).*(7.0./4.0e+1)+cos(theta2+pi./2.0).*(7.0./4.0e+1)+3.0./2.5e+1).^2).*(5.0./3.0))+atan2(sin(theta1-pi./2.0).*(-7.0./4.0e+1)-sin(theta2+pi./2.0).*(7.0./4.0e+1),abs(cos(theta1-pi./2.0).*(7.0./4.0e+1)+cos(theta2+pi./2.0).*(7.0./4.0e+1)+3.0./2.5e+1))+6.012387278395987e-2).*(-3.328470665197855e-1)+cos(theta2+pi./2.0).*(7.0./4.0e+1)+3.0./5.0e+1).^2+(sin(acos(sqrt((sin(theta1-pi./2.0).*(7.0./4.0e+1)+sin(theta2+pi./2.0).*(7.0./4.0e+1)).^2+abs(cos(theta1-pi./2.0).*(7.0./4.0e+1)+cos(theta2+pi./2.0).*(7.0./4.0e+1)+3.0./2.5e+1).^2).*(5.0./3.0))+atan2(sin(theta1-pi./2.0).*(-7.0./4.0e+1)-sin(theta2+pi./2.0).*(7.0./4.0e+1),abs(cos(theta1-pi./2.0).*(7.0./4.0e+1)+cos(theta2+pi./2.0).*(7.0./4.0e+1)+3.0./2.5e+1))+6.012387278395987e-2).*3.328470665197855e-1+sin(theta2+pi./2.0).*(7.0./4.0e+1)).^2);
end

== matlab function RaibertControl/Final/AK90-M1/MATLAB Function ==
  data: tff_cmd input; q_cmd input; w_cmd input; Kp_cmd input; Kd_cmd input; q input; t output; w input
function t = PD(tff_cmd,q_cmd,w_cmd,Kp_cmd,Kd_cmd,q,w)
t = Kp_cmd*(q_cmd - q) + Kd_cmd*(w_cmd - w) + tff_cmd;

%function t = PD(cmd,q,w)
%t = cmd.Kp*(cmd.q - q) + cmd.Kd*(cmd.w - w) + cmd.tff;

== matlab function RaibertControl/Final/Planarising Boom/MATLAB Function ==
  data: roll_q input; roll_w input; pitch_q input; pitch_w input; pitch_b input; yaw_q input; state output Bus: BodyState; yaw_w input; yaw_b input; y_body output
function [state,y_body] = boom_state(roll_q, roll_w, pitch_q, pitch_w, pitch_b, yaw_q, yaw_w, yaw_b)
yawRadius = 2.575; % m
pitchRadius = 2.493; % m
pitchHeightOffset = 0.101; % m

state.x = yawRadius * yaw_q;
state.dx = yawRadius * yaw_w;
state.ddx = yawRadius * yaw_b;

state.y = pitchRadius * sin(pitch_q) + pitchHeightOffset;
state.dy = pitchRadius * cos(pitch_q) * pitch_w;
state.ddy = pitchRadius * cos(pitch_q) * pitch_b - pitchRadius * sin(pitch_q) * pitch_w * pitch_w;

state.r = roll_q;
state.dr = roll_w;

y_body =  pitchRadius * sin(pitch_q) + pitchHeightOffset;
end

== matlab function RaibertControl/Final/Impedance Control/MATLAB Function ==
  data: theta1 input; JT11 output; theta2 input; JT12 output; JT21 output; JT22 output
function [JT11,JT12,JT21,JT22] = Jacobian_Transpose(theta1,theta2)
%JACOBIAN_TRANSPOSE
%    [JT11,JT12,JT21,JT22] = JACOBIAN_TRANSPOSE(THETA1,THETA2)

%    This function was generated by the Symbolic Math Toolbox version 8.6.
%    17-May-2022 09:32:09

t2 = pi./2.0;
t3 = -t2;
t4 = t2+theta2;
t5 = t3+theta1;
t6 = cos(t4);
t7 = sin(t4);
t8 = cos(t5);
t9 = sin(t5);
t10 = t6.*(7.0./4.0e+1);
t11 = t7.*(7.0./4.0e+1);
t14 = t7.*1.75e-1i;
t12 = t8.*(7.0./4.0e+1);
t13 = t9.*(7.0./4.0e+1);
t15 = t9.*1.75e-1i;
t16 = -t14;
t17 = -t15;
t18 = t11+t13;
t20 = t10+t12+3.0./2.5e+1;
t19 = t18.^2;
t21 = abs(t20);
t22 = sign(t20);
t29 = t6.*t18.*(7.0./2.0e+1);
t31 = t8.*t18.*(7.0./2.0e+1);
t23 = t21.^2;
t24 = 1.0./t21;
t26 = t19.*(2.5e+1./9.0);
t35 = t16+t17+t21;
t42 = t7.*t21.*t22.*(7.0./2.0e+1);
t43 = t9.*t21.*t22.*(7.0./2.0e+1);
t25 = 1.0./t23;
t27 = -t26;
t28 = t23.*(2.5e+1./9.0);
t32 = t10.*t24;
t33 = t12.*t24;
t34 = t19+t23;
t36 = angle(t35);
t44 = -t42;
t45 = -t43;
t30 = -t28;
t37 = 1.0./t34;
t38 = sqrt(t34);
t48 = t11.*t18.*t22.*t25;
t49 = t13.*t18.*t22.*t25;
t50 = t29+t44;
t51 = t31+t45;
t39 = 1.0./t38;
t40 = t38.*(5.0./3.0);
t46 = t27+t30+1.0;
t52 = t32+t48;
t53 = t33+t49;
t41 = acos(t40);
t47 = 1.0./sqrt(t46);
t66 = t23.*t37.*t52;
t67 = t23.*t37.*t53;
t54 = t36+t41+6.012387278395987e-2;
t68 = t39.*t47.*t50.*(5.0./6.0);
t69 = t39.*t47.*t51.*(5.0./6.0);
t55 = cos(t54);
t56 = sin(t54);
t73 = t66+t68;
t74 = t67+t69;
t57 = t55.*3.328470665197855e-1;
t58 = t56.*3.328470665197855e-1;
t77 = t55.*t73.*(-3.328470665197855e-1);
t59 = -t57;
t60 = t11+t58;
t75 = t57.*t73;
t76 = t58.*t73;
t79 = t10+t77;
t61 = t60.^2;
t62 = t10+t59+3.0./5.0e+1;
t78 = t11+t76;
t63 = t62.^2;
t64 = 1.0./t62;
t65 = 1.0./t63;
t70 = t61+t63;
t71 = 1.0./t70;
t72 = 1.0./sqrt(t70);
JT11 = t72.*(t55.*t60.*t74.*6.65694133039571e-1+t56.*t62.*t74.*6.65694133039571e-1).*(-1.0./2.0);
if nargout > 1
    JT12 = t63.*t71.*(t57.*t64.*t74-t56.*t60.*t65.*t74.*3.328470665197855e-1);
end
if nargout > 2
    JT21 = (t72.*(t60.*t79.*2.0-t62.*t78.*2.0))./2.0;
end
if nargout > 3
    JT22 = -t63.*t71.*(t64.*t79+t60.*t65.*t78);
end

== matlab function RaibertControl/Final/Impedance Control1/MATLAB Function ==
  data: theta1 input; JT11 output; theta2 input; JT12 output; JT21 output; JT22 output
function [JT11,JT12,JT21,JT22] = Jacobian_Transpose(theta1,theta2)
%JACOBIAN_TRANSPOSE
%    [JT11,JT12,JT21,JT22] = JACOBIAN_TRANSPOSE(THETA1,THETA2)

%    This function was generated by the Symbolic Math Toolbox version 8.6.
%    17-May-2022 09:32:09

t2 = pi./2.0;
t3 = -t2;
t4 = t2+theta2;
t5 = t3+theta1;
t6 = cos(t4);
t7 = sin(t4);
t8 = cos(t5);
t9 = sin(t5);
t10 = t6.*(7.0./4.0e+1);
t11 = t7.*(7.0./4.0e+1);
t14 = t7.*1.75e-1i;
t12 = t8.*(7.0./4.0e+1);
t13 = t9.*(7.0./4.0e+1);
t15 = t9.*1.75e-1i;
t16 = -t14;
t17 = -t15;
t18 = t11+t13;
t20 = t10+t12+3.0./2.5e+1;
t19 = t18.^2;
t21 = abs(t20);
t22 = sign(t20);
t29 = t6.*t18.*(7.0./2.0e+1);
t31 = t8.*t18.*(7.0./2.0e+1);
t23 = t21.^2;
t24 = 1.0./t21;
t26 = t19.*(2.5e+1./9.0);
t35 = t16+t17+t21;
t42 = t7.*t21.*t22.*(7.0./2.0e+1);
t43 = t9.*t21.*t22.*(7.0./2.0e+1);
t25 = 1.0./t23;
t27 = -t26;
t28 = t23.*(2.5e+1./9.0);
t32 = t10.*t24;
t33 = t12.*t24;
t34 = t19+t23;
t36 = angle(t35);
t44 = -t42;
t45 = -t43;
t30 = -t28;
t37 = 1.0./t34;
t38 = sqrt(t34);
t48 = t11.*t18.*t22.*t25;
t49 = t13.*t18.*t22.*t25;
t50 = t29+t44;
t51 = t31+t45;
t39 = 1.0./t38;
t40 = t38.*(5.0./3.0);
t46 = t27+t30+1.0;
t52 = t32+t48;
t53 = t33+t49;
t41 = acos(t40);
t47 = 1.0./sqrt(t46);
t66 = t23.*t37.*t52;
t67 = t23.*t37.*t53;
t54 = t36+t41+6.012387278395987e-2;
t68 = t39.*t47.*t50.*(5.0./6.0);
t69 = t39.*t47.*t51.*(5.0./6.0);
t55 = cos(t54);
t56 = sin(t54);
t73 = t66+t68;
t74 = t67+t69;
t57 = t55.*3.328470665197855e-1;
t58 = t56.*3.328470665197855e-1;
t77 = t55.*t73.*(-3.328470665197855e-1);
t59 = -t57;
t60 = t11+t58;
t75 = t57.*t73;
t76 = t58.*t73;
t79 = t10+t77;
t61 = t60.^2;
t62 = t10+t59+3.0./5.0e+1;
t78 = t11+t76;
t63 = t62.^2;
t64 = 1.0./t62;
t65 = 1.0./t63;
t70 = t61+t63;
t71 = 1.0./t70;
t72 = 1.0./sqrt(t70);
JT11 = t72.*(t55.*t60.*t74.*6.65694133039571e-1+t56.*t62.*t74.*6.65694133039571e-1).*(-1.0./2.0);
if nargout > 1
    JT12 = t63.*t71.*(t57.*t64.*t74-t56.*t60.*t65.*t74.*3.328470665197855e-1);
end
if nargout > 2
    JT21 = (t72.*(t60.*t79.*2.0-t62.*t78.*2.0))./2.0;
end
if nargout > 3
    JT22 = -t63.*t71.*(t64.*t79+t60.*t65.*t78);
end

== matlab function RaibertControl/Final/AK90-M2/MATLAB Function ==
  data: tff_cmd input; q_cmd input; w_cmd input; Kp_cmd input; Kd_cmd input; q input; t output; w input
function t = PD(tff_cmd,q_cmd,w_cmd,Kp_cmd,Kd_cmd,q,w)
t = Kp_cmd*(q_cmd - q) + Kd_cmd*(w_cmd - w) + tff_cmd;

%function t = PD(cmd,q,w)
%t = cmd.Kp*(cmd.q - q) + cmd.Kd*(cmd.w - w) + cmd.tff;

== matlab function RaibertControl/Final/AK90-M4/MATLAB Function ==
  data: tff_cmd input; q_cmd input; w_cmd input; Kp_cmd input; Kd_cmd input; q input; t output; w input
function t = PD(tff_cmd,q_cmd,w_cmd,Kp_cmd,Kd_cmd,q,w)
t = Kp_cmd*(q_cmd - q) + Kd_cmd*(w_cmd - w) + tff_cmd;

%function t = PD(cmd,q,w)
%t = cmd.Kp*(cmd.q - q) + cmd.Kd*(cmd.w - w) + cmd.tff;

== matlab function RaibertControl/Final/AK90-M3/MATLAB Function ==
  data: tff_cmd input; q_cmd input; w_cmd input; Kp_cmd input; Kd_cmd input; q input; t output; w input
function t = PD(tff_cmd,q_cmd,w_cmd,Kp_cmd,Kd_cmd,q,w)
t = Kp_cmd*(q_cmd - q) + Kd_cmd*(w_cmd - w) + tff_cmd;

%function t = PD(cmd,q,w)
%t = cmd.Kp*(cmd.q - q) + cmd.Kd*(cmd.w - w) + cmd.tff;

== matlab function RaibertControl/Final/Impedance Control/MATLAB Function3 ==
  data: F_push input; tau1 output; r input; phi input; r_ref input; phi_ref input; dr input; dphi input; JT11 input; JT12 input; JT21 input; JT22 input; tau2 output
function [tau1,tau2]  = Controller(F_push,r,phi,r_ref,phi_ref,dr,dphi,JT11,JT12,JT21,JT22)
    dr_ref = 0.0;
    dphi_ref = 0.0;
    JT = [JT11,JT12;JT21,JT22];
    Kp_r = 500;  
    Kp_phi = 50;  
    Kd_r = 10;  
    Kd_phi = 1; 
    
    E = [r_ref - r; phi_ref - phi];
    dE = [dr_ref - dr; dphi_ref - dphi];
    
    if r<0.39
        wr = Kp_r*E(1) + Kd_r*dE(1) + F_push;
        wphi = Kp_phi*E(2) + Kd_phi*dE(2);
    else 
        wr = Kp_r*E(1) + Kd_r*dE(1);
        wphi = Kp_phi*E(2) + Kd_phi*dE(2);
    end
    
    w = [wr;wphi];
    tau = JT*w;
    tau1 = tau(1);
    tau2 = tau(2);
    
end
